simulink model "svpwm"  (R2014a)
settings: Solver=ode45  StartTime=0.0  StopTime=3  RelTol=1e-3
libraries: powerlib x3
settings Model: Creator=Administrator  LastModifiedBy=Administrator
settings DataIOCC: InspectSignalLogs=on

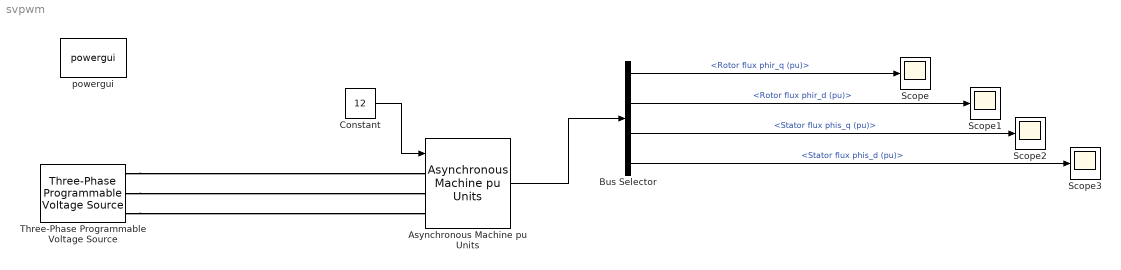
== system svpwm ==
  Asynchronous Machine pu Units : powerlib/Machines/Asynchronous Machine pu Units  PresetModel=No  MechanicalLoad=Torque Tm  ShowDetailedParameters=on  RotorType=Squirrel-cage  ReferenceFrame=Rotor  Units=pu  MeasurementBus=off  NominalParameters=[3730 460 60]  Stator=[0.01965 0.0397]  Rotor=[0.01909 0.0397]  Cage1=[0.01909 0.0397]  Cage2=[0.01909 0.0397]  Lm=1.354  Mechanical=[0.09526 0.05479 2]  PolePairs=2  InitialConditions="[ 1,0   0,0,0   0,0,0 ]"  SimulateSaturation=off  Saturation="[0.212,0.4201,0.8125,1.0979,1.4799,2.2457,3.2586,4.5763,6.4763 ;   0.5,0.7,0.9,1,1.1,1.2 ,1.3,1.4,1.5]"  LoadFlowParameters=0  TsPowergui=0  TsBlock=0.00001  IterativeModel=Trapezoidal non iterative  Pmec=0.0000000001
  Bus Selector : BusSelector  OutputSignals=Rotor measurements.Rotor flux phir_q (pu),Rotor measurements.Rotor flux phir_d (pu),Stator measurements.Stator flux phis_q (pu),Stator measurements.Stator flux phis_d (pu)
  Constant : Constant  Value=12
  Scope{,1..3} (4 alike) : Scope
      Scope settings: YMin=-0.0008  YMax=0.0008
      Scope1 settings: YMin=-0.0005  YMax=0.0005
      Scope2 settings: YMin=-0.225  YMax=0.225  SaveName=ScopeData2
      Scope3 settings: YMin=-0.0008  YMax=0.0008  SaveName=ScopeData3
  Three-Phase Programmable Voltage Source : powerlib/Electrical Sources/Three-Phase Programmable Voltage Source  PositiveSequence="[100  0 60]"  VariationEntity=None  VariationType=Table of time-amplitude pairs  VariationTypeAlt=Step  VariationStep=0.5  VariationRate=10  VariationMagnitude=0.3  VariationFrequency=2  VariationTiming=[1 2]  VariationPhaseA=off  Amplitudes=[1 0.8 1.2 1.0]  TimeValues=[0 0.1 0.15 0.2]  HarmonicGeneration=off  HarmonicA=[3 0.2 -25 0]  HarmonicB=[2 0.15 35 2]  Timing="[0.05  3]"  BusType=swing  Pref=0  Qref=0  Qmin=-inf  Qmax=inf
  powergui : powerlib/powergui  Priority=1  SimulationMode=Continuous  SolverType=Tustin  SampleTime=50e-6  frequency=60  SPID=off  DisableSnubberDevices=off  DisableRonSwitches=off  DisableVfSwitches=off  SwTol=0  Interpol=off  DisplayEquations=off  Ts=0  methode=off  frequencyindice=60  Pbase=100e6  ErrMax=1e-4  Iterations=50  UnitsV=kV  UnitsW=MW  FunctionMessages=off  echomessages=off  HookPort=off  EnableUseOfTLC=off  x0status=blocks  RestoreLinks=warning  ResistiveCurrentMeasurement=off  Frange=[0:2:500]  Ylog=off  Xlog=on  ShowGrid=off  save=off  variable=ZData  structure=0  ZoomFFT=off  StartTime=0.0  cycles=1  DisplayStyle=1  fundamental=60  FreqAxis=off  MaxFrequency=1000  frequencyindicesteady=1  RmsSteady=1  display=off
  wires:
  Asynchronous Machine pu Units/1 -> Bus Selector/1
  Bus Selector/1 -> Scope/1  "<Rotor flux phir_q (pu)>"
  Bus Selector/2 -> Scope1/1  "<Rotor flux phir_d (pu)>"
  Constant/1 -> Asynchronous Machine pu Units/1
  Bus Selector/3 -> Scope2/1  "<Stator flux phis_q (pu)>"
  Bus Selector/4 -> Scope3/1  "<Stator flux phis_d (pu)>"
  connections:
  Three-Phase Programmable Voltage Source/RConn1 -- Asynchronous Machine pu Units/LConn1
  Three-Phase Programmable Voltage Source/RConn2 -- Asynchronous Machine pu Units/LConn2
  Three-Phase Programmable Voltage Source/RConn3 -- Asynchronous Machine pu Units/LConn3
